simulink model "mi_modelo_dtmf"  (R2025b)
settings: Solver=VariableStepAuto  StartTime=0.0  StopTime=0.25  RelTol=1e-3
settings Model: Creator=johnd  LastModifiedBy=johnd

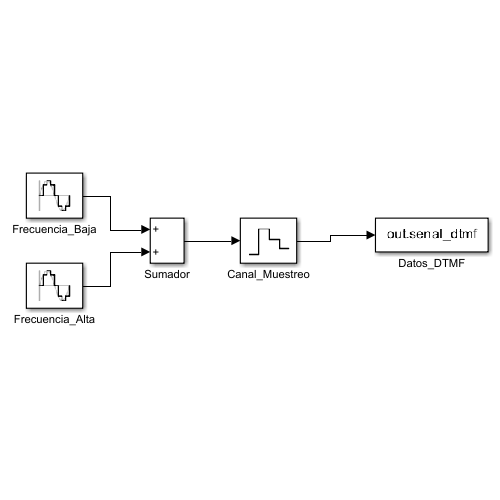
[thumbnail: Simulink's stored preview of the top-level diagram]
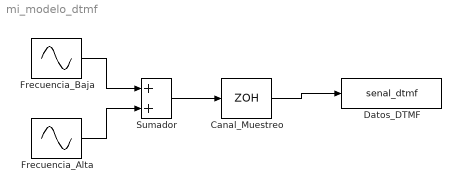
== system mi_modelo_dtmf ==
  Canal_Muestreo : ZeroOrderHold  SampleTime=0.000125
  Datos_DTMF : ToWorkspace  VariableName=senal_dtmf  SaveFormat=Timeseries  SampleTime=-1
  Frecuencia_Alta : Sin  Frequency=2*pi*1336  SampleTime=0.000125
  Frecuencia_Baja : Sin  Frequency=2*pi*770  SampleTime=0.000125
  Sumador : Sum
  wires:
  Frecuencia_Baja/1 -> Sumador/1
  Frecuencia_Alta/1 -> Sumador/2
  Sumador/1 -> Canal_Muestreo/1
  Canal_Muestreo/1 -> Datos_DTMF/1
